simulink model "model_V16a"  (Simulink 9.2)
settings: Solver=FixedStepAuto  StartTime=0.0  StopTime=30  FixedStep=0.01  RelTol=1e-2  AbsTol=1e-2
values from neighbouring files (symbols this model uses):
  control = ans'    [anim.m]
  vent = [vvent(i,2);vvent(i,3);vvent(i,4)]    [anim.m]
undefined symbols (not defined in the file or in its folder): dynamique, imu, vr
libraries: simulink x3
settings Model: Creator=pmorin  LastModifiedBy=idris  ExtModeAutoUpdateStatusClock=off
settings SolverCC: AutoScaleAbsTol=off  AutoInsertRateTranBlk=on
settings DataIOCC: SignalLoggingSaveFormat=Dataset
settings OptimizationCC: BooleanDataType=off  ExpressionDepthLimit=2147483647  InitFltsAndDblsToZero=on
settings DebuggingCC: SaveWithParameterizedLinksMsg=none  SignalResolutionControl=TryResolveAllWithWarning  MultiTaskDSMMsg=warning  MultiTaskCondExecSysMsg=none  SFExecutionAtInitializationDiag=warning
settings HardwareCC: TargetUnknown=on
settings GRTTargetCC: ModelReferenceCompliant=off  CompOptLevelCompliant=off  MatFileLogging=off

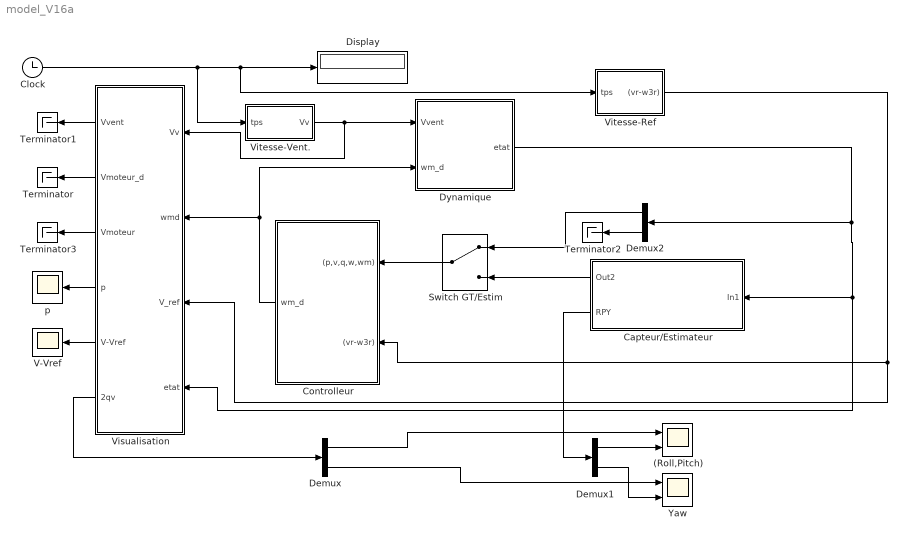
== system model_V16a ==
  (Roll,Pitch) : Scope  NumInputPorts=2
  Capteur/Estimateur : Subsystem  TreatAsAtomicUnit=on
  Clock : Clock
  Controlleur : Subsystem
  Demux : Demux  Outputs=[2; 1]
  Demux1 : Demux  Outputs=[2;1]
  Demux2 : Demux  Outputs=[17 3]
  Display : Display
  Dynamique : Subsystem  mask{init=[0.5;0.5;1;0;0;0;sqrt(1-0^2);-0;0;0;0;0;0.3;600;600;600;600]}
      mask prompts: init "Initial values"
  Switch GT/Estim : ManualSwitch
  Terminator{,1..3} (4 alike) : Terminator
  V-Vref : Scope
  Visualisation : Subsystem
  Vitesse-Ref : Subsystem  mask{choix_traj=Vitesse périodique}
      mask prompts: choix_traj "trajectoire de reference"
      mask TypeOptions choix_traj: Vitesse nulle | Vitesse constante | Vitesse périodique | Autre
  Vitesse-Vent. : Subsystem  mask{choix_traj=sans vent}
      mask prompts: choix_traj "trajectoire de reference"
      mask TypeOptions choix_traj: sans vent | vent constant | vent periodique | vent rafale | vent general
  Yaw : Scope  NumInputPorts=2
  p : Scope
  wires:
  Clock/1 -> Vitesse-Vent./1(tps), Vitesse-Ref/1(tps), Display/1
  Vitesse-Vent./1(Vv) -> Visualisation/1(Vv), Dynamique/1(Vvent)
  Controlleur/1(wm_d) -> Dynamique/2(wm_d), Visualisation/2(wmd)
  Visualisation/4(p) -> p/1
  Visualisation/5(V-Vref) -> V-Vref/1
  Visualisation/3("Vmoteur ") -> Terminator3/1
  Vitesse-Ref/1((vr-w3r)) -> Visualisation/3(V_ref), Controlleur/2((vr-w3r))
  Visualisation/2(Vmoteur_d) -> Terminator/1
  Visualisation/1(Vvent) -> Terminator1/1
  Dynamique/1(etat) -> Demux2/1, Visualisation/4(etat), Capteur/Estimateur/1(In1)
  Visualisation/6(2qv) -> Demux/1
  Demux/1 -> (Roll,Pitch)/1
  Demux1/1 -> (Roll,Pitch)/2
  Demux1/2 -> Yaw/2
  Capteur/Estimateur/2(RPY) -> Demux1/1
  Capteur/Estimateur/1(Out2) -> Switch GT/Estim/2
  Switch GT/Estim/1 -> Controlleur/1((p,v,q,w,wm))
  Demux2/1 -> Switch GT/Estim/1
  Demux2/2 -> Terminator2/1
  Demux/2 -> Yaw/1

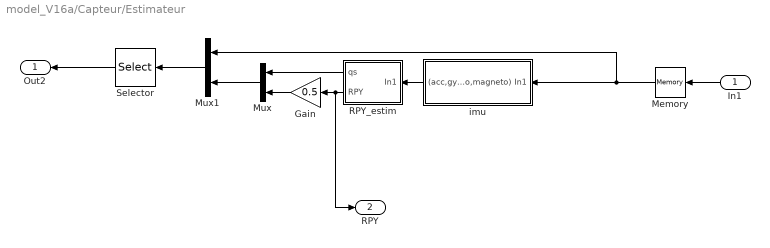
== system model_V16a/Capteur/Estimateur ==
  In1 : Inport
  Gain : Gain  Gain=0.5
  Memory : Memory  InheritSampleTime=on
  Mux : Mux  Inputs=2
  Mux1 : Mux  Inputs=2
  RPY_estim : Subsystem  TreatAsAtomicUnit=on
  Selector : Selector  InputPortWidth=24  IndexOptions=Index vector (dialog)  Indices=[1 2 3 4 5 6 21 22 23 24 11 12 13 14 15 16 17]  OutputSizes=1
  imu : Subsystem  TreatAsAtomicUnit=on
  Out2 : Outport
  RPY : Outport  Port=2
  wires:
  RPY_estim/1(qs) -> Mux/1
  imu/1((acc,gyro,magneto)) -> RPY_estim/1(In1)
  Memory/1 -> Mux1/1, imu/1(In1)
  Gain/1 -> Mux/2
  RPY_estim/2(RPY) -> RPY/1, Gain/1
  In1/1 -> Memory/1
  Mux/1 -> Mux1/2
  Mux1/1 -> Selector/1
  Selector/1 -> Out2/1

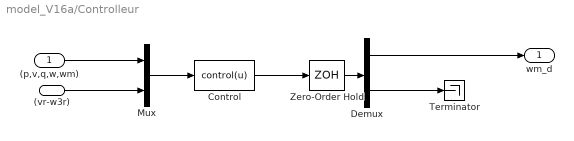
== system model_V16a/Controlleur ==
  (p,v,q,w,wm) : Inport
  (vr-w3r) : Inport  Port=2
  Control : MATLABFcn  MATLABFcn=control(u)  OutputDimensions=7
  Demux : Demux  Outputs=2
  Mux : Mux  Inputs=2
  Terminator : Terminator
  Zero-Order Hold : ZeroOrderHold  SampleTime=0.01
  wm_d : Outport
  wires:
  Control/1 -> Zero-Order Hold/1
  Mux/1 -> Control/1
  (p,v,q,w,wm)/1 -> Mux/1
  Zero-Order Hold/1 -> Demux/1
  Demux/1 -> wm_d/1
  Demux/2 -> Terminator/1
  (vr-w3r)/1 -> Mux/2

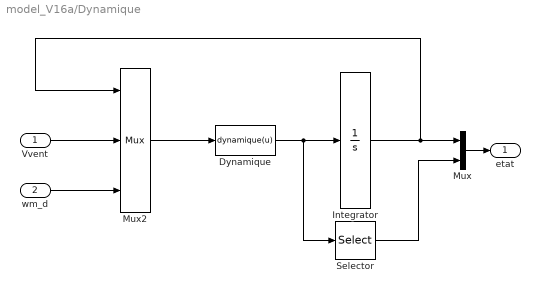
== system model_V16a/Dynamique ==
  Vvent : Inport
  wm_d : Inport  Port=2
  Dynamique : MATLABFcn  MATLABFcn=dynamique(u)  OutputDimensions=17
  Integrator : Integrator  InitialCondition=init
  Mux : Mux  Inputs=2
  Mux2 : Mux  Inputs=[17 3 4]
  Selector : Selector  InputPortWidth=17  IndexOptions=Index vector (dialog)  Indices=[4 5 6]  OutputSizes=1
  etat : Outport
  wires:
  Vvent/1 -> Mux2/2
  wm_d/1 -> Mux2/3
  Mux2/1 -> Dynamique/1
  Dynamique/1 -> Selector/1, Integrator/1
  Mux/1 -> etat/1
  Selector/1 -> Mux/2
  Integrator/1 -> Mux2/1, Mux/1

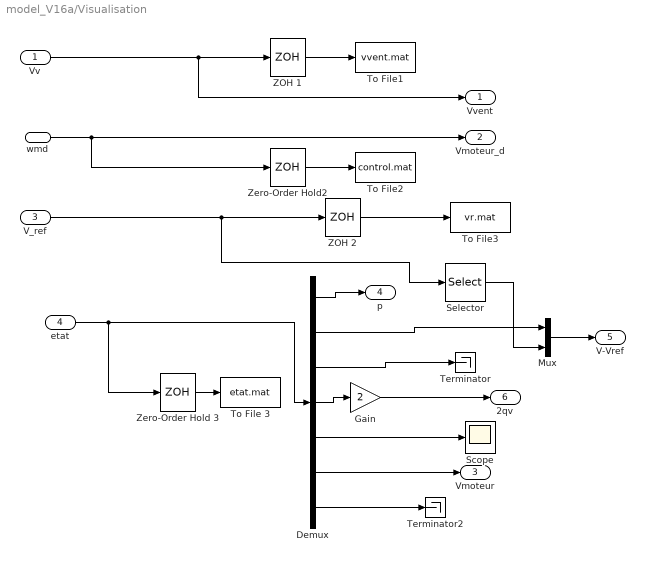
== system model_V16a/Visualisation ==
  Vv : Inport
  wmd : Inport  Port=2
  V_ref : Inport  Port=3
  etat : Inport  Port=4
  Demux : Demux  Outputs=[3 3 1 3 3 4 3]
  Gain : Gain  Gain=2
  Mux : Mux  Inputs=2
  Scope : Scope
  Selector : Selector  InputPortWidth=4  IndexOptions=Index vector (dialog)  Indices=[1 2 3]  OutputSizes=1
  Terminator : Terminator
  Terminator2 : Terminator
  To File 3 : ToFile  Filename=etat.mat
  To File1 : ToFile  Filename=vvent.mat
  To File2 : ToFile  Filename=control.mat
  To File3 : ToFile  Filename=vr.mat
  ZOH 1 : ZeroOrderHold  SampleTime=0.02
  "ZOH 2 " : ZeroOrderHold  SampleTime=0.4
  Zero-Order Hold 3 : ZeroOrderHold  SampleTime=0.02
  Zero-Order Hold2 : ZeroOrderHold  SampleTime=0.4
  Vvent : Outport
  Vmoteur_d : Outport  Port=2
  "Vmoteur " : Outport  Port=3
  p : Outport  Port=4
  V-Vref : Outport  Port=5
  2qv : Outport  Port=6
  wires:
  Zero-Order Hold 3/1 -> To File 3/1
  Vv/1 -> Vvent/1, ZOH 1/1
  etat/1 -> Zero-Order Hold 3/1, Demux/1
  Zero-Order Hold2/1 -> To File2/1
  ZOH 1/1 -> To File1/1
  Demux/1 -> p/1
  wmd/1 -> Vmoteur_d/1, Zero-Order Hold2/1
  Gain/1 -> 2qv/1
  Demux/4 -> Gain/1
  Demux/3 -> Terminator/1
  Demux/6 -> "Vmoteur "/1
  V_ref/1 -> Selector/1, "ZOH 2 "/1
  "ZOH 2 "/1 -> To File3/1
  Demux/2 -> Mux/1
  Mux/1 -> V-Vref/1
  Selector/1 -> Mux/2
  Demux/5 -> Scope/1
  Demux/7 -> Terminator2/1

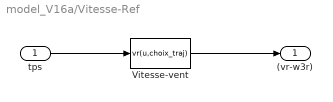
== system model_V16a/Vitesse-Ref ==
  tps : Inport
  Vitesse-vent : MATLABFcn  MATLABFcn=vr(u,choix_traj)  OutputDimensions=4
  (vr-w3r) : Outport
  wires:
  Vitesse-vent/1 -> (vr-w3r)/1
  tps/1 -> Vitesse-vent/1

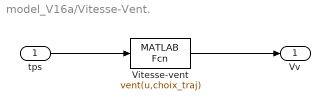
== system model_V16a/Vitesse-Vent. ==
  tps : Inport
  Vitesse-vent : MATLABFcn  MATLABFcn=vent(u,choix_traj)  OutputDimensions=3
  Vv : Outport
  wires:
  Vitesse-vent/1 -> Vv/1
  tps/1 -> Vitesse-vent/1

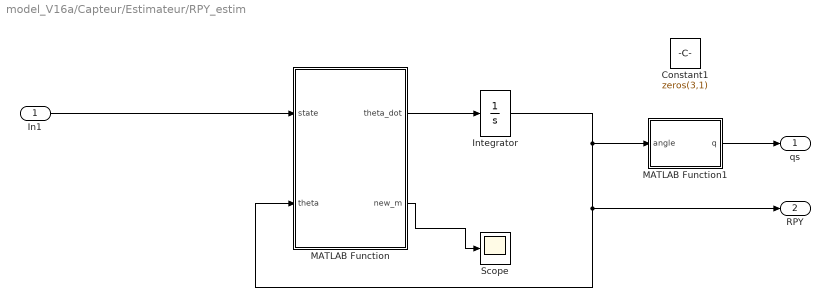
== system model_V16a/Capteur/Estimateur/RPY_estim ==
  In1 : Inport
  Constant1 : Constant  Value=zeros(3,1)
  Integrator : Integrator
  MATLAB Function : MATLAB Function  TreatAsAtomicUnit=on
  MATLAB Function1 : MATLAB Function  TreatAsAtomicUnit=on
  Scope : Scope
  qs : Outport
  RPY : Outport  Port=2
  wires:
  In1/1 -> MATLAB Function/1(state)
  Integrator/1 -> MATLAB Function/2(theta), RPY/1, MATLAB Function1/1(angle)
  MATLAB Function1/1(q) -> qs/1
  MATLAB Function/2(new_m) -> Scope/1
  MATLAB Function/1(theta_dot) -> Integrator/1

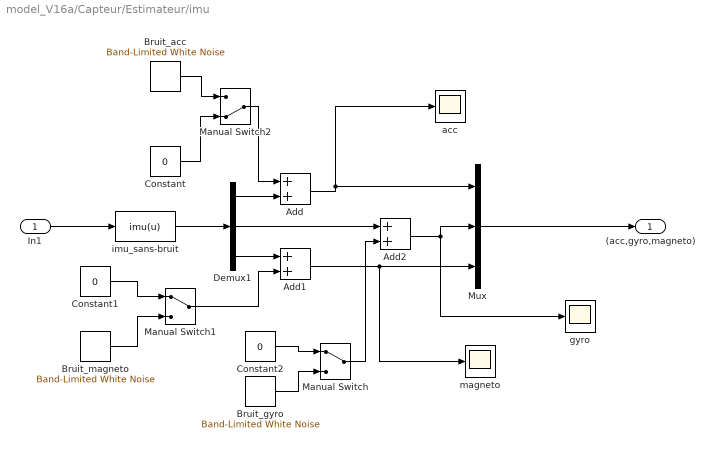
== system model_V16a/Capteur/Estimateur/imu ==
  In1 : Inport
  Add : Sum
  Add1 : Sum
  Add2 : Sum
  Bruit_acc : simulink/Sources/Band-Limited White Noise  Cov=[0.1]  Ts=0.01  seed=[23341;12025;15426]
  Bruit_gyro : simulink/Sources/Band-Limited White Noise  Cov=[0.001]  Ts=0.01  seed=[21241;15625;17326]
  Bruit_magneto : simulink/Sources/Band-Limited White Noise  Cov=[1e-10]  Ts=0.01  seed=[9821;13120;22478]
  Constant : Constant  Value=0
  Constant1 : Constant  Value=0
  Constant2 : Constant  Value=0
  Demux1 : Demux  Outputs=3
  Manual Switch : ManualSwitch
  Manual Switch1 : ManualSwitch
  Manual Switch2 : ManualSwitch  CurrentSetting=0
  Mux : Mux  Inputs=3
  acc : Scope
  gyro : Scope
  imu_sans-bruit : MATLABFcn  MATLABFcn=imu(u)  OutputDimensions=9
  "magneto " : Scope
  (acc,gyro,magneto) : Outport
  wires:
  In1/1 -> imu_sans-bruit/1
  Add/1 -> acc/1, Mux/1
  imu_sans-bruit/1 -> Demux1/1
  Demux1/1 -> Add/2
  Demux1/3 -> Add1/1
  Demux1/2 -> Add2/1
  Add2/1 -> gyro/1, Mux/2
  Add1/1 -> "magneto "/1, Mux/3
  Mux/1 -> (acc,gyro,magneto)/1
  Bruit_gyro/1 -> Manual Switch/2
  Constant2/1 -> Manual Switch/1
  Manual Switch/1 -> Add2/2
  Bruit_magneto/1 -> Manual Switch1/2
  Constant1/1 -> Manual Switch1/1
  Manual Switch1/1 -> Add1/2
  Manual Switch2/1 -> Add/1
  Constant/1 -> Manual Switch2/2
  Bruit_acc/1 -> Manual Switch2/1

== matlab function Capteur//Estimateur/RPY_estim/MATLAB Function1 ==
  data: angle input double; q output double
function q = fcn(angle)
theta = zeros(1,3);
theta(1)= angle(1);
theta(2)= angle(2);
theta(3)= angle(3);
theta
truc = (theta(1)^2 + theta(2)^2 + theta(3)^2)/4;

qs = 1 - truc;
u = sqrt(abs(qs));

q = u;

== matlab function Capteur//Estimateur/RPY_estim/MATLAB Function ==
  data: state input double; theta_dot output double; theta input double; new_m output double
function [theta_dot, new_m] = estim_lin(state, theta)
g = 9.81;
a_m = state(1:3);
w_m = state(4:6);
m_m = state(7:9);
m_i_1 = 4.7e-5*cos(65*pi/180);
m_m_bar = m_m - (m_m*(a_m/g)')*a_m/g;

theta_dot = zeros(1,3);
k1 = 0.01;
k2 = 0.01;
k3 = 0.500;
theta_dot(1)= w_m(1) - k1*(theta(1) + (a_m(2)/g));
theta_dot(2)= w_m(2) - k2*(theta(1) - (a_m(2)/g));
new_m = m_m_bar/m_i_1;

e_2 = [0; 1; 0];
theta_dot(3)= w_m(3) - k3*(theta(3) + (new_m')*e_2);

end
